simulink model "Analysis_model_MOD"  (R2025b)
settings: Solver=ode2  StartTime=0.0  StopTime=Tf  FixedStep=Tstep  RelTol=1e-3
values from neighbouring files (symbols this model uses):
  Km = 1300    [Stabilization.m]    (also in Stabilization_Mod.m = 1)
  Kp = (2*W_cl*Zeta_cl*Time_const - 1)/Km    [Stabilization_Mod.m]
  Sim_disturbance_amplitude = 8    [Stabilization_Mod.m]
  Sim_disturbance_freq = pi    (= 3.14159265359)    [Stabilization_Mod.m]
  Sim_saturation_neg = -20    [Stabilization_Mod.m]
  Sim_saturation_pos = 20    [Stabilization_Mod.m]
  Time_const = 0.0573    [Stabilization_Mod.m]
  Tsample = 0.005    [Stabilization_Mod.m]
undefined symbols (not defined in the file or in its folder): DiscIntNeverNeededParam
settings Model: Creator=GILBERT  LastModifiedBy=GILBERT

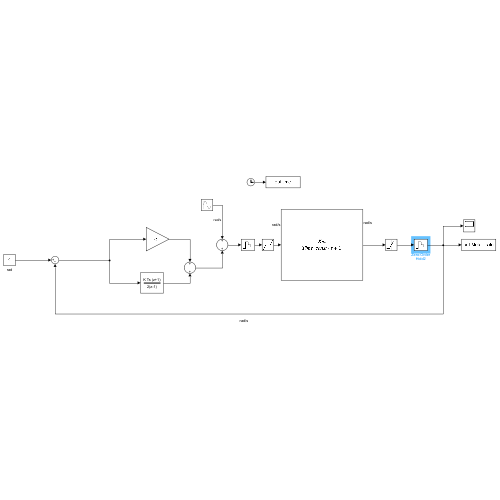
[thumbnail: Simulink's stored preview of the top-level diagram]
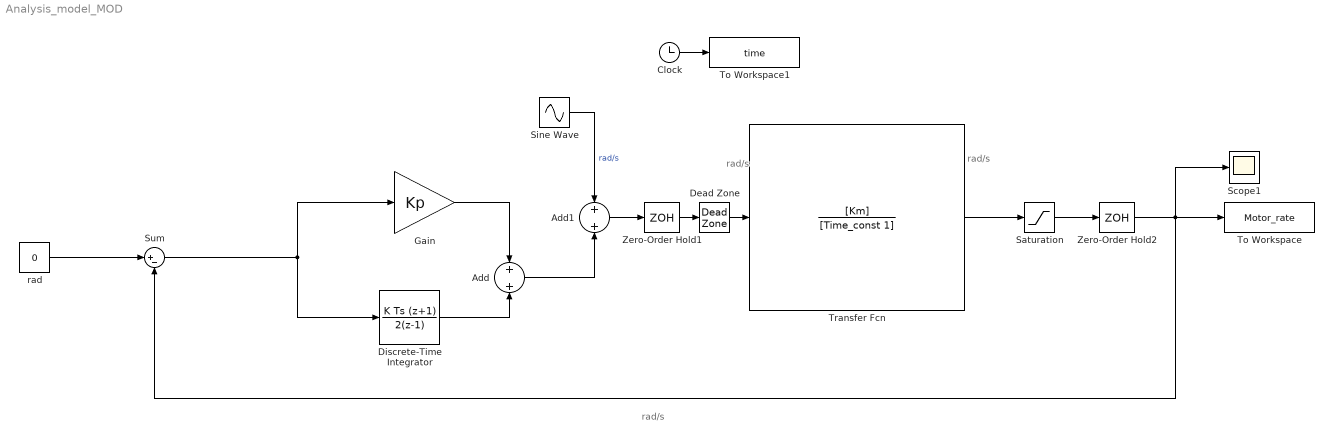
== system Analysis_model_MOD ==
  note: rad/s
  note: rad/s
  note: rad/s
  Add : Sum
  Add1 : Sum
  Clock : Clock
  Dead Zone : DeadZone  LowerValue=Sim_deadZone_start  UpperValue=Sim_deadZone_final
  Discrete-Time Integrator : DiscreteIntegrator  IntegratorMethod=Integration: Trapezoidal  gainval=Ki  SampleTime=Tsample  ICPrevOutput=DiscIntNeverNeededParam  ICPrevScaledInput=DiscIntNeverNeededParam
  Gain : Gain  Gain=Kp
  Saturation : Saturate  UpperLimit=Sim_saturation_pos  LowerLimit=Sim_saturation_neg
  Scope1 : Scope
      settings: ActiveDisplayYMinimum=-1.1644474527973081  ActiveDisplayYMaximum=1.0939827146871717
  Sine Wave : Sin  Amplitude=Sim_disturbance_amplitude  Frequency=Sim_disturbance_freq  SampleTime=Tsample
  Sum : Sum  Inputs=|+-
  To Workspace : ToWorkspace  VariableName=Motor_rate  SaveFormat=Timeseries  SampleTime=-1
  To Workspace1 : ToWorkspace  VariableName=time  SaveFormat=Timeseries  SampleTime=-1
  Transfer Fcn : TransferFcn  Numerator=[Km]  Denominator=[Time_const 1]
  Zero-Order Hold1 : ZeroOrderHold  SampleTime=Tsample
  Zero-Order Hold2 : ZeroOrderHold  SampleTime=Tsample
  rad : Constant  Value=0
  wires:
  Gain/1 -> Add/1
  Add/1 -> Add1/2
  Sine Wave/1 -> Add1/1  "rad/s"
  Sum/1 -> Discrete-Time Integrator/1, Gain/1
  rad/1 -> Sum/1
  Add1/1 -> Zero-Order Hold1/1
  Discrete-Time Integrator/1 -> Add/2
  Zero-Order Hold1/1 -> Dead Zone/1
  Dead Zone/1 -> Transfer Fcn/1
  Saturation/1 -> Zero-Order Hold2/1
  Zero-Order Hold2/1 -> To Workspace/1, Scope1/1, Sum/2
  Clock/1 -> To Workspace1/1
  Transfer Fcn/1 -> Saturation/1
